simulink model "ControllerWrapper"  (R2026a)
settings: Solver=FixedStepAuto
undefined symbols (not defined in the file): controllerParams, final_track_index
libraries: simulink x1
settings Model: Creator=rayyu  LastModifiedBy=rayyu
settings RTWCC: SystemTargetFile=ert.tlc  Description=Embedded Coder
settings ERTTargetCC: GenerateSampleERTMain=on

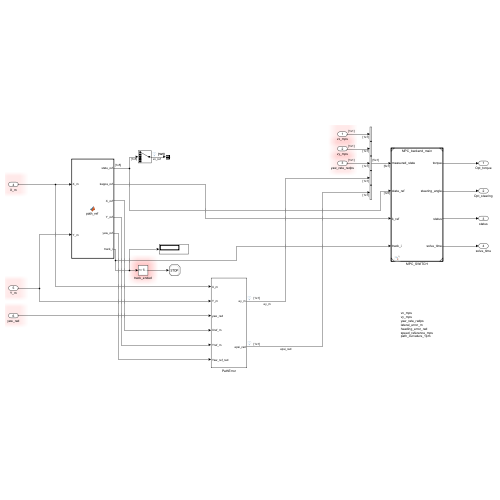
[thumbnail: Simulink's stored preview of the top-level diagram]
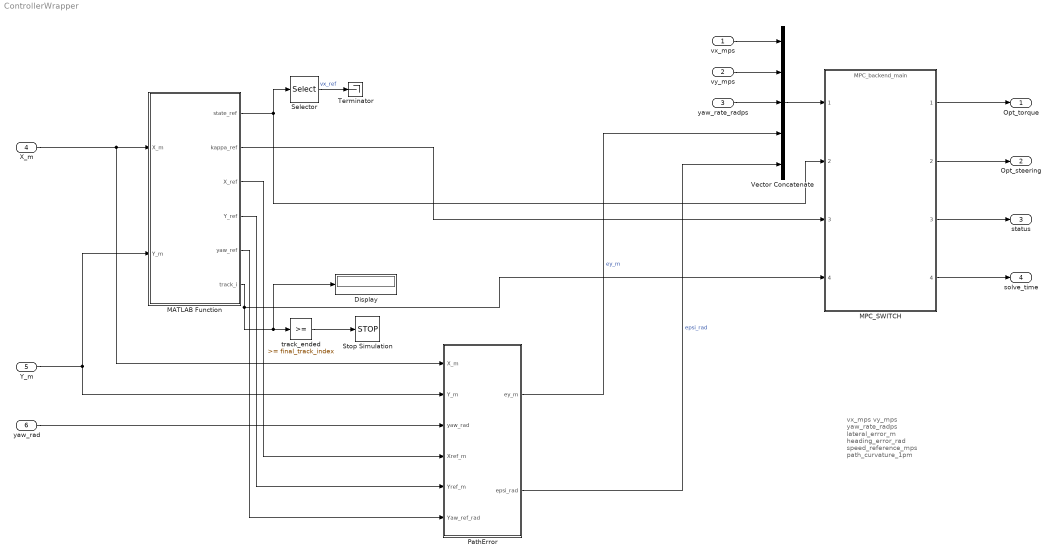
== system ControllerWrapper ==
  note: vx_mps
      | vy_mps
      | yaw_rate_radps
      | lateral_error_m
      | heading_error_rad
      | speed_reference_mps
      | path_curvature_1pm
  vx_mps : Inport  SampleTime=controllerParams.Ts_s
  vy_mps : Inport  Port=2  SampleTime=controllerParams.Ts_s
  yaw_rate_radps : Inport  Port=3  SampleTime=controllerParams.Ts_s
  X_m : Inport  Port=4  SampleTime=controllerParams.Ts_s
  Y_m : Inport  Port=5  SampleTime=controllerParams.Ts_s
  yaw_rad : Inport  Port=6  SampleTime=controllerParams.Ts_s
  Display : Display
  MATLAB Function : MATLAB Function  TreatAsAtomicUnit=on
  MPC_SWITCH : ModelReference  ModelNameDialog=MPC_backend_main.slx  SimulationMode=Normal  ModelReferenceVersion=1.80
  PathError : Subsystem
  Selector : Selector  InputPortWidth=5  IndexOptions=Index vector (dialog)  Indices=1  OutputSizes=1
  Stop Simulation : Stop
  Terminator : Terminator
  Vector Concatenate : Concatenate  NumInputs=5
  track_ended : simulink/Logic and Bit Operations/Compare To Constant  relop=>=  const=final_track_index  OutDataTypeStr=boolean
  Opt_torque : Outport
  Opt_steering : Outport  Port=2
  status : Outport  Port=3
  solve_time : Outport  Port=4
  wires:
  vx_mps/1 -> Vector Concatenate/1
  vy_mps/1 -> Vector Concatenate/2
  yaw_rate_radps/1 -> Vector Concatenate/3
  PathError/1(ey_m) -> Vector Concatenate/4  "ey_m"
  PathError/2(epsi_rad) -> Vector Concatenate/5  "epsi_rad"
  Vector Concatenate/1 -> MPC_SWITCH/1
  MPC_SWITCH/3 -> status/1
  MPC_SWITCH/2 -> Opt_steering/1
  MPC_SWITCH/1 -> Opt_torque/1
  MATLAB Function/1(state_ref) -> MPC_SWITCH/2, Selector/1
  MATLAB Function/4(Y_ref) -> PathError/5(Yref_m)
  MATLAB Function/5(yaw_ref) -> PathError/6(Yaw_ref_rad)
  MATLAB Function/3(X_ref) -> PathError/4(Xref_m)
  X_m/1 -> PathError/1(X_m), MATLAB Function/1(X_m)
  Y_m/1 -> MATLAB Function/2(Y_m), PathError/2(Y_m)
  yaw_rad/1 -> PathError/3(yaw_rad)
  MATLAB Function/2(kappa_ref) -> MPC_SWITCH/3
  Selector/1 -> Terminator/1  "vx_ref"
  MPC_SWITCH/4 -> solve_time/1
  MATLAB Function/6(track_i) -> MPC_SWITCH/4, Display/1, track_ended/1
  track_ended/1 -> Stop Simulation/1

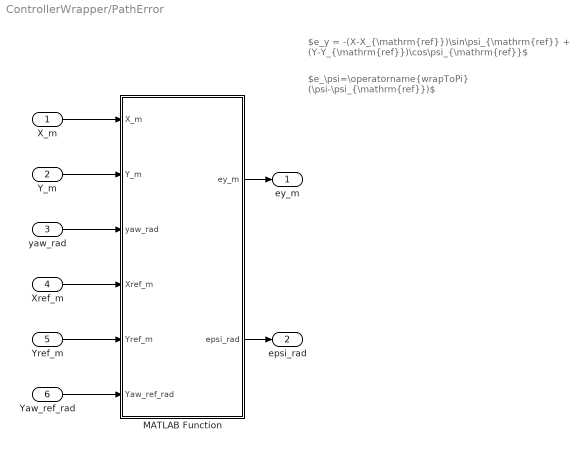
== system ControllerWrapper/PathError ==
  note: $e_\psi=\operatorname{wrapToPi} (\psi-\psi_{\mathrm{ref}})$
  note: $e_y = -(X-X_{\mathrm{ref}})\sin\psi_{\mathrm{ref}} + (Y-Y_{\mathrm{ref}})\cos\psi_{\mathrm{ref}}$
  X_m : Inport
  Y_m : Inport  Port=2
  yaw_rad : Inport  Port=3
  Xref_m : Inport  Port=4
  Yref_m : Inport  Port=5
  Yaw_ref_rad : Inport  Port=6
  MATLAB Function : MATLAB Function  TreatAsAtomicUnit=on
  ey_m : Outport
  epsi_rad : Outport  Port=2
  wires:
  X_m/1 -> MATLAB Function/1(X_m)
  Y_m/1 -> MATLAB Function/2(Y_m)
  yaw_rad/1 -> MATLAB Function/3(yaw_rad)
  Xref_m/1 -> MATLAB Function/4(Xref_m)
  Yref_m/1 -> MATLAB Function/5(Yref_m)
  Yaw_ref_rad/1 -> MATLAB Function/6(Yaw_ref_rad)
  MATLAB Function/1(ey_m) -> ey_m/1
  MATLAB Function/2(epsi_rad) -> epsi_rad/1

== matlab function ControllerWrapper/MATLAB Function ==
  data: X_m input; state_ref output size=[1 5]; Y_m input; kappa_ref output; X_ref output; Y_ref output; yaw_ref output; track_ref_table parameter; track_i output
function [state_ref, ...
          kappa_ref, ...
          X_ref, ...
          Y_ref, ...
          yaw_ref, ...
          track_i ...
          ] = ...
          path_ref( ...
              X_m, ...
              Y_m,...
              track_ref_table)
% track_reference_table columns:
% 1: s
% 2: X
% 3: Y
% 4: psi
% 5: kappa
% 6: vx reference
% 7: yaw-rate reference

%% Find closest track point
distanceSquared = ...
    (track_ref_table(:,2) - X_m).^2 + ...
    (track_ref_table(:,3) - Y_m).^2;

[~, track_i] = min(distanceSquared);


%% Extract local path reference

X_ref = ...
    track_ref_table(track_i, 2);

Y_ref = ...
    track_ref_table(track_i, 3);

yaw_ref = ...
    track_ref_table(track_i, 4);

kappa_ref = ...
    track_ref_table(track_i, 5);

vx_reference = ...
    track_ref_table(track_i, 6);

yaw_rate_reference = ...
    track_ref_table(track_i, 7);

%% Construct MPC state reference

state_ref = zeros(1,5);

state_ref(1) = vx_reference;
state_ref(2) = 0;
state_ref(3) = yaw_rate_reference;
state_ref(4) = 0;
state_ref(5) = 0;

end

== matlab function ControllerWrapper/PathError/MATLAB Function ==
  data: X_m input; ey_m output; Y_m input; yaw_rad input; Xref_m input; Yref_m input; Yaw_ref_rad input; epsi_rad output
function [ey_m, epsi_rad] = ...
    PathError( ...
    X_m, ...
    Y_m, ...
    yaw_rad, ...
    Xref_m, ...
    Yref_m, ...
    Yaw_ref_rad)
% Position relative to the selected reference-path point
deltaX = X_m - Xref_m;
deltaY = Y_m - Yref_m;
% Signed lateral error
ey_m = ...
    -deltaX * sin(Yaw_ref_rad) + ...
    deltaY * cos(Yaw_ref_rad);
% Wrap heading error to [-pi, pi]
epsi_rad = atan2( ...
    sin(yaw_rad - Yaw_ref_rad), ...
    cos(yaw_rad - Yaw_ref_rad));

end
